simulink model "Task1"  (R2024a)
settings: Solver=VariableStepAuto  StartTime=0.0  StopTime=10.0  RelTol=1e-3
settings Model: Creator=artemzmailov  LastModifiedBy=artemzmailov

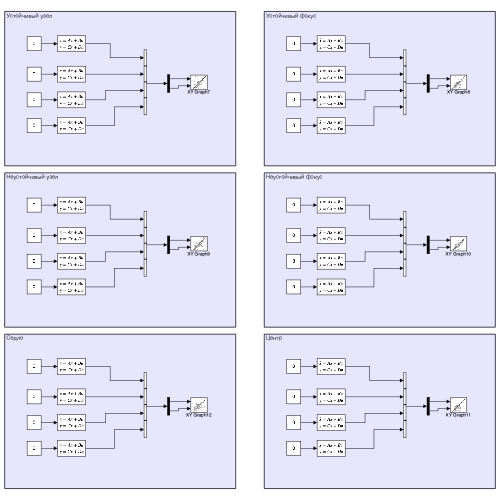
[thumbnail: Simulink's stored preview of the top-level diagram]
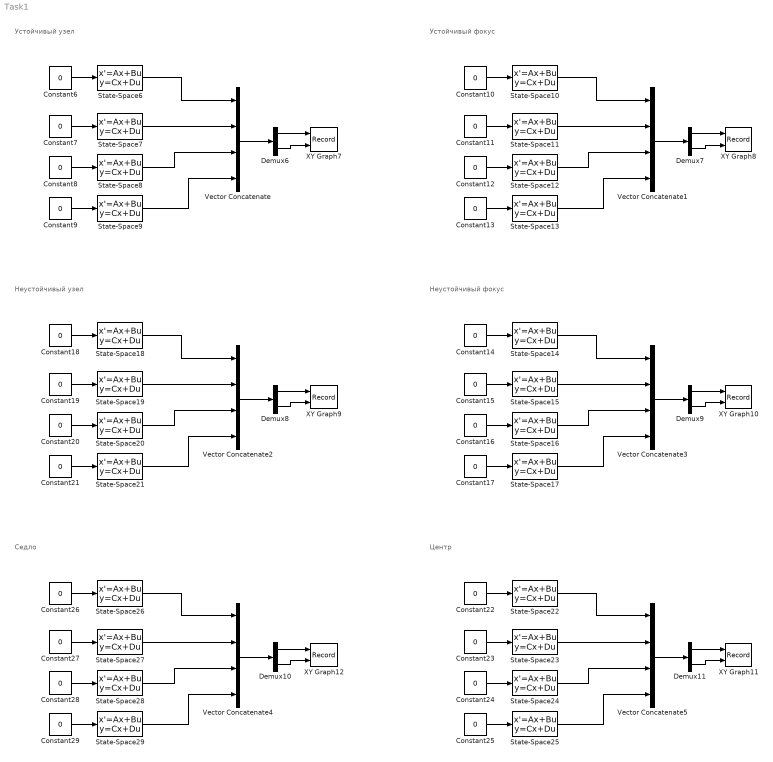
== system Task1 ==
  note: Устойчивый узел
  note: Устойчивый фокус
  note: Неустойчивый узел
  note: Неустойчивый фокус
  note: Седло
  note: Центр
  Constant{6..29} (24 alike) : Constant  Value=0
  Demux{6..11} (6 alike) : Demux  Outputs=2
  State-Space10 : StateSpace  A=[-1 -1; 2 -2]  B=[0;0]  C=[1 0; 0 1]  D=[0;0]  InitialCondition=[1;1]
  State-Space11 : StateSpace  A=[-1 0; 0 -2]  B=[0;0]  C=[1 0; 0 1]  D=[0;0]  InitialCondition=[-1;1]
  State-Space12 : StateSpace  A=[-1 0; 0 -2]  B=[0;0]  C=[1 0; 0 1]  D=[0;0]  InitialCondition=[3;-3]
  State-Space13 : StateSpace  A=[-1 0; 0 -2]  B=[0;0]  C=[1 0; 0 1]  D=[0;0]  InitialCondition=[-1;-1]
  State-Space14 : StateSpace  A=[1 -1; 2 2]  B=[0;0]  C=[1 0; 0 1]  D=[0;0]  InitialCondition=[1;1]
  State-Space15 : StateSpace  A=[1 -1; 2 2]  B=[0;0]  C=[1 0; 0 1]  D=[0;0]  InitialCondition=[-1;1]
  State-Space16 : StateSpace  A=[1 -1; 2 2]  B=[0;0]  C=[1 0; 0 1]  D=[0;0]  InitialCondition=[3;-3]
  State-Space17 : StateSpace  A=[1 -1; 2 2]  B=[0;0]  C=[1 0; 0 1]  D=[0;0]  InitialCondition=[-1;-1]
  State-Space18 : StateSpace  A=[1 0; 0 2]  B=[0;0]  C=[1 0; 0 1]  D=[0;0]  InitialCondition=[1;1]
  State-Space19 : StateSpace  A=[1 0; 0 2]  B=[0;0]  C=[1 0; 0 1]  D=[0;0]  InitialCondition=[-1;1]
  State-Space20 : StateSpace  A=[1 0; 0 2]  B=[0;0]  C=[1 0; 0 1]  D=[0;0]  InitialCondition=[0.5;-0.5]
  State-Space21 : StateSpace  A=[1 0; 0 2]  B=[0;0]  C=[1 0; 0 1]  D=[0;0]  InitialCondition=[-1;-1]
  State-Space22 : StateSpace  A=[0 -1; 1 0]  B=[0;0]  C=[1 0; 0 1]  D=[0;0]  InitialCondition=[1;1]
  State-Space23 : StateSpace  A=[0 -1; 1 0]  B=[0;0]  C=[1 0; 0 1]  D=[0;0]  InitialCondition=[-1;1]
  State-Space24 : StateSpace  A=[0 -1; 1 0]  B=[0;0]  C=[1 0; 0 1]  D=[0;0]  InitialCondition=[3;-3]
  State-Space25 : StateSpace  A=[0 -1; 1 0]  B=[0;0]  C=[1 0; 0 1]  D=[0;0]  InitialCondition=[-1;-1]
  State-Space26 : StateSpace  A=[1 0; 0 -2]  B=[0;0]  C=[1 0; 0 1]  D=[0;0]  InitialCondition=[1;1]
  State-Space27 : StateSpace  A=[1 0; 0 -2]  B=[0;0]  C=[1 0; 0 1]  D=[0;0]  InitialCondition=[-1;1]
  State-Space28 : StateSpace  A=[1 0; 0 -2]  B=[0;0]  C=[1 0; 0 1]  D=[0;0]  InitialCondition=[3;-3]
  State-Space29 : StateSpace  A=[1 0; 0 -2]  B=[0;0]  C=[1 0; 0 1]  D=[0;0]  InitialCondition=[-1;-1]
  State-Space6 : StateSpace  A=[-1 0; 0 -2]  B=[0;0]  C=[1 0; 0 1]  D=[0;0]  InitialCondition=[1;1]
  State-Space7 : StateSpace  A=[-1 0; 0 -2]  B=[0;0]  C=[1 0; 0 1]  D=[0;0]  InitialCondition=[-1;1]
  State-Space8 : StateSpace  A=[-1 0; 0 -2]  B=[0;0]  C=[1 0; 0 1]  D=[0;0]  InitialCondition=[3;-3]
  State-Space9 : StateSpace  A=[-1 0; 0 -2]  B=[0;0]  C=[1 0; 0 1]  D=[0;0]  InitialCondition=[-1;-1]
  Vector Concatenate{,1..5} (6 alike) : Concatenate  NumInputs=4
  XY Graph10 : Record  FileSettingsInternal="{\"entries\":[{\"content\":{\"excelSettings\":{\"content\":{},\"type\":\"Streamout.ExcelSettings\"}},\"type\":\"Streamout.FileSettingStorage\",\"uuid\":\"\"}],\"packageUris\":[\"http:\\/\\/schema.mathworks.com\\/mf0\\/streamout_blocks\\/R2020a\"],\"version\":\"1.0\"}"  Layout=[1 1]  SignalsInternal="{\"entries\":[{\"content\":{},\"type\":\"RecordBlkView.InputSignals\",\"uuid\":\"\"}],\"packageUris\":[\"http:\\/\\/schema.mathworks.com\\/mf0\\/streamout_blocks\\/R2020a\"],\"version\":\"1.0\"}"  VisualizationBindings="{\"xyplotplugin\":{\"info\":[{\"series\":[{\"bindingParametersList\":[{\"parameter\":\"X-Axis\",\"signalID\":2387,\"signalName\":\"Demux9:1(1)\"},{\"parameter\":\"Y-Axis\",\"signalID\":2392,\"signalName\":\"Demux9:2(1)\"}],\"seriesID\":0},{\"bindingParametersList\":[{\"parameter\":\"X-Axis\",\"signalID\":2442,\"signalName\":\"Demux9:1(2)\"},{\"parameter\":\"Y-Axis\",\"signalID\":2445,\"signalName\":\"Demux9:2(2)\"}],\"seriesID\":1},{\"bindingParametersList\":[{\"parameter\":\"X-Axis\",\"signalID\":2443,\"signalName\":\"Demux9:1(3)\"},{\"parameter\":\"Y-Axis\",\"signalID\":2446,\"signalName\":\"Demux9:2(3)\"}],\"seriesID\":2},{\"bindingParametersList\":[{\"parameter\":\"X-Axis\",\"signalID\":2444,\"signalName\":\"Demux9:1(4)\"},{\"parameter\":\"Y-Axis\",\"signalID\":2447,\"signalName\":\"Demux9:2(4)\"}],\"seriesID\":3}],\"subplotID\":1}]}}"  CompatibilityTag=XY
  XY Graph11 : Record  FileSettingsInternal="{\"entries\":[{\"content\":{\"excelSettings\":{\"content\":{},\"type\":\"Streamout.ExcelSettings\"}},\"type\":\"Streamout.FileSettingStorage\",\"uuid\":\"\"}],\"packageUris\":[\"http:\\/\\/schema.mathworks.com\\/mf0\\/streamout_blocks\\/R2020a\"],\"version\":\"1.0\"}"  Layout=[1 1]  SignalsInternal="{\"entries\":[{\"content\":{},\"type\":\"RecordBlkView.InputSignals\",\"uuid\":\"\"}],\"packageUris\":[\"http:\\/\\/schema.mathworks.com\\/mf0\\/streamout_blocks\\/R2020a\"],\"version\":\"1.0\"}"  VisualizationBindings="{\"xyplotplugin\":{\"info\":[{\"series\":[{\"bindingParametersList\":[{\"parameter\":\"X-Axis\",\"signalID\":2407,\"signalName\":\"Demux11:1(1)\"},{\"parameter\":\"Y-Axis\",\"signalID\":2412,\"signalName\":\"Demux11:2(1)\"}],\"seriesID\":0},{\"bindingParametersList\":[{\"parameter\":\"X-Axis\",\"signalID\":2454,\"signalName\":\"Demux11:1(2)\"},{\"parameter\":\"Y-Axis\",\"signalID\":2457,\"signalName\":\"Demux11:2(2)\"}],\"seriesID\":1},{\"bindingParametersList\":[{\"parameter\":\"X-Axis\",\"signalID\":2455,\"signalName\":\"Demux11:1(3)\"},{\"parameter\":\"Y-Axis\",\"signalID\":2458,\"signalName\":\"Demux11:2(3)\"}],\"seriesID\":2},{\"bindingParametersList\":[{\"parameter\":\"X-Axis\",\"signalID\":2456,\"signalName\":\"Demux11:1(4)\"},{\"parameter\":\"Y-Axis\",\"signalID\":2459,\"signalName\":\"Demux11:2(4)\"}],\"seriesID\":3}],\"subplotID\":1}]}}"  CompatibilityTag=XY
  XY Graph12 : Record  FileSettingsInternal="{\"entries\":[{\"content\":{\"excelSettings\":{\"content\":{},\"type\":\"Streamout.ExcelSettings\"}},\"type\":\"Streamout.FileSettingStorage\",\"uuid\":\"\"}],\"packageUris\":[\"http:\\/\\/schema.mathworks.com\\/mf0\\/streamout_blocks\\/R2020a\"],\"version\":\"1.0\"}"  Layout=[1 1]  SignalsInternal="{\"entries\":[{\"content\":{},\"type\":\"RecordBlkView.InputSignals\",\"uuid\":\"\"}],\"packageUris\":[\"http:\\/\\/schema.mathworks.com\\/mf0\\/streamout_blocks\\/R2020a\"],\"version\":\"1.0\"}"  VisualizationBindings="{\"xyplotplugin\":{\"info\":[{\"series\":[{\"bindingParametersList\":[{\"parameter\":\"X-Axis\",\"signalID\":2417,\"signalName\":\"Demux10:1(1)\"},{\"parameter\":\"Y-Axis\",\"signalID\":2422,\"signalName\":\"Demux10:2(1)\"}],\"seriesID\":0},{\"bindingParametersList\":[{\"parameter\":\"X-Axis\",\"signalID\":2460,\"signalName\":\"Demux10:1(2)\"},{\"parameter\":\"Y-Axis\",\"signalID\":2463,\"signalName\":\"Demux10:2(2)\"}],\"seriesID\":1},{\"bindingParametersList\":[{\"parameter\":\"X-Axis\",\"signalID\":2461,\"signalName\":\"Demux10:1(3)\"},{\"parameter\":\"Y-Axis\",\"signalID\":2464,\"signalName\":\"Demux10:2(3)\"}],\"seriesID\":2},{\"bindingParametersList\":[{\"parameter\":\"X-Axis\",\"signalID\":2462,\"signalName\":\"Demux10:1(4)\"},{\"parameter\":\"Y-Axis\",\"signalID\":2465,\"signalName\":\"Demux10:2(4)\"}],\"seriesID\":3}],\"subplotID\":1}]}}"  CompatibilityTag=XY
  XY Graph7 : Record  FileSettingsInternal="{\"entries\":[{\"content\":{\"excelSettings\":{\"content\":{},\"type\":\"Streamout.ExcelSettings\"}},\"type\":\"Streamout.FileSettingStorage\",\"uuid\":\"\"}],\"packageUris\":[\"http:\\/\\/schema.mathworks.com\\/mf0\\/streamout_blocks\\/R2020a\"],\"version\":\"1.0\"}"  Layout=[1 1]  SignalsInternal="{\"entries\":[{\"content\":{},\"type\":\"RecordBlkView.InputSignals\",\"uuid\":\"\"}],\"packageUris\":[\"http:\\/\\/schema.mathworks.com\\/mf0\\/streamout_blocks\\/R2020a\"],\"version\":\"1.0\"}"  VisualizationBindings="{\"xyplotplugin\":{\"info\":[{\"series\":[{\"bindingParametersList\":[{\"parameter\":\"X-Axis\",\"signalID\":2427,\"signalName\":\"Demux6:1(1)\"},{\"parameter\":\"Y-Axis\",\"signalID\":2432,\"signalName\":\"Demux6:2(1)\"},{\"parameter\":\"X-Axis\",\"signalID\":2427,\"signalName\":\"Demux6:1(1)\"},{\"parameter\":\"Y-Axis\",\"signalID\":2432,\"signalName\":\"Demux6:2(1)\"},{\"parameter\":\"X-Axis\",\"signalID\":2427,\"signalName\":\"Demux6:1(1)\"},{\"parameter\":\"Y-Axis\",\"signalID\":2432,\"signalName\":\"Demux6:2(1)\"},{\"parameter\":\"X-Axis\",\"signalID\":2427,\"signalName\":\"Demux6:1(1)\"},{\"parameter\":\"Y-Axis\",\"signalID\":2432,\"signalName\":\"Demux6:2(1)\"},{\"parameter\":\"X-Axis\",\"signalID\":2427,\"signalName\":\"Demux6:1(1)\"},{\"parameter\":\"Y-Axis\",\"signalID\":2432,\"signalName\":\"Demux6:2(1)\"},{\"parameter\":\"X-Axis\",\"signalID\":2427,\"signalName\":\"Demux6:1(1)\"},{\"parameter\":\"Y-Axis\",\"signalID\":2432,\"signalName\":\"Demux6:2(1)\"},{\"parameter\":\"X-Axis\",\"signalID\":2427,\"signalName\":\"Demux6:1(1)\"},{\"parameter\":\"Y-Axis\",\"signalID\":2432,\"signalName\":\"Demux6:2(1)\"},{\"parameter\":\"X-Axis\",\"signalID\":2427,\"signalName\":\"Demux6:1(1)\"},{\"parameter\":\"Y-Axis\",\"signalID\":2432,\"signalName\":\"Demux6:2(1)\"},{\"parameter\":\"X-Axis\",\"signalID\":2427,\"signalName\":\"Demux6:1(1)\"},{\"parameter\":\"Y-Axis\",\"signalID\":2432,\"signalName\":\"Demux6:2(1)\"},{\"parameter\":\"X-Axis\",\"signalID\":2427,\"signalName\":\"Demux6:1(1)\"},{\"parameter\":\"Y-Axis\",\"signalID\":2432,\"signalName\":\"Demux6:2(1)\"},{\"parameter\":\"X-Axis\",\"signalID\":2427,\"signalName\":\"Demux6:1(1)\"},{\"parameter\":\"Y-Axis\",\"signalID\":2432,\"signalName\":\"Demux6:2(1)\"},{\"parameter\":\"X-Axis\",\"signalID\":2427,\"signalName\":\"Demux6:1(1)\"},{\"parameter\":\"Y-Axis\",\"signalID\":2432,\"signalName\":\"Demux6:2(1)\"},{\"parameter\":\"X-Axis\",\"signalID\":2427,\"signalName\":\"Demux6:1(1)\"},{\"parameter\":\"Y-Axis\",\"signalID\":2432,\"signalName\":\"Demux6:2(1)\"},{\"parameter\":\"X-Axis\",\"signalID\":2427,\"signalName\":\"Demux6:1(1)\"},{\"parameter\":\"Y-Axis\",\"signalID\":2432,\"signalName\":\"Demux6:2(1)\"},{\"parameter\":\"X-Axis\",\"signalID\":2427,\"signalName\":\"Demux6:1(1)\"},{\"parameter\":\"Y-Axis\",\"signalID\":2432,\"signalName\":\"Demux6:2(1)\"},{\"parameter\":\"X-Axis\",\"signalID\":2427,\"signalName\":\"Demux6:1(1)\"},{\"parameter\":\"Y-Axis\",\"signalID\":2432,\"signalName\":\"Demux6:2(1)\"}],\"seriesID\":0},{\"bindingParametersList\":[{\"parameter\":\"X-Axis\",\"signalID\":2466,\"signalName\":\"Demux6:1(2)\"},{\"parameter\":\"Y-Axis\",\"signalID\":2469,\"signalName\":\"Demux6:2(2)\"},{\"parameter\":\"X-Axis\",\"signalID\":2466,\"signalName\":\"Demux6:1(2)\"},{\"parameter\":\"Y-Axis\",\"signalID\":2469,\"signalName\":\"Demux6:2(2)\"},{\"parameter\":\"X-Axis\",\"signalID\":2466,\"signalName\":\"Demux6:1(2)\"},{\"parameter\":\"Y-Axis\",\"signalID\":2469,\"signalName\":\"Demux6:2(2)\"},{\"parameter\":\"X-Axis\",\"signalID\":2466,\"signalName\":\"Demux6:1(2)\"},{\"parameter\":\"Y-Axis\",\"signalID\":2469,\"signalName\":\"Demux6:2(2)\"},{\"parameter\":\"X-Axis\",\"signalID\":2466,\"signalName\":\"Demux6:1(2)\"},{\"parameter\":\"Y-Axis\",\"signalID\":2469,\"signalName\":\"Demux6:2(2)\"},{\"parameter\":\"X-Axis\",\"signalID\":2466,\"signalName\":\"Demux6:1(2)\"},{\"parameter\":\"Y-Axis\",\"signalID\":2469,\"signalName\":\"Demux6:2(2)\"},{\"parameter\":\"X-Axis\",\"signalID\":2466,\"signalName\":\"Demux6:1(2)\"},{\"parameter\":\"Y-Axis\",\"signalID\":2469,\"signalName\":\"Demux6:2(2)\"},{\"parameter\":\"X-Axis\",\"signalID\":2466,\"signalName\":\"Demux6:1(2)\"},{\"parameter\":\"Y-Axis\",\"signalID\":2469,\"signalName\":\"Demux6:2(2)\"},{\"parameter\":\"X-Axis\",\"signalID\":2466,\"signalName\":\"Demux6:1(2)\"},{\"parameter\":\"Y-Axis\",\"signalID\":2469,\"signalName\":\"Demux6:2(2)\"},{\"parameter\":\"X-Axis\",\"signalID\":2466,\"signalName\":\"Demux6:1(2)\"},{\"parameter\":\"Y-Axis\",\"signalID\":2469,\"signalName\":\"Demux6:2(2)\"},{\"parameter\":\"X-Axis\",\"signalID\":2466,\"signalName\":\"Demux6:1(2)\"},{\"parameter\":\"Y-Axis\",\"signalID\":2469,\"signalName\":\"Demux6:2(2)\"},{\"parameter\":\"X-Axis\",\"signalID\":2466,\"signalName\":\"Demux6:1(2)\"},{\"parameter\":\"Y-Axis\",\"signalID\":2469,\"signalName\":\"Demux6:2(2)\"},{\"parameter\":\"X-Axis\",\"signalID\":2466,\"signalName\":\"Demux6:1(2)\"},{\"parameter\":\"Y-Axis\",\"signalID\":2469,\"signalName\":\"Demux6:2(2)\"},{\"parameter\":\"X-Axis\",\"signalID\":2466,\"signalName\":\"Demux6:1(2)\"},{\"parameter\":\"Y-Axis\",\"signalID\":2469,\"signalName\":\"Demux6:2(2)\"},{\"parameter\":\"X-Axis\",\"signalID\":2466,\"signalName\":\"Demux6:1(2)\"},{\"parameter\":\"Y-Axis\",\"signalID\":2469,\"signalName\":\"Demux6:2(2)\"}],\"seriesID\":1},{\"bindingParametersList\":[{\"parameter\":\"X-Axis\",\"signalID\":2467,\"signalName\":\"Demux6:1(3)\"},{\"parameter\":\"Y-Axis\",\"signalID\":2470,\"signalName\":\"Demux6:2(3)\"},{\"parameter\":\"X-Axis\",\"signalID\":2467,\"signalName\":\"Demux6:1(3)\"},{\"parameter\":\"Y-Axis\",\"signalID\":2470,\"signalName\":\"Demux6:2(3)\"},{\"parameter\":\"X-Axis\",\"signalID\":2467,\"signalName\":\"Demux6:1(3)\"},{\"parameter\":\"Y-Axis\",\"signalID\":2470,\"signalName\":\"Demux6:2(3)\"},{\"parameter\":\"X-Axis\",\"signalID\":2467,\"signalName\":\"Demux6:1(3)\"},{\"parameter\":\"Y-Axis\",\"signalID\":2470,\"signalName\":\"Demux6:2(3)\"},{\"parameter\":\"X-Axis\",\"signalID\":2467,\"signalName\":\"Demux6:1(3)\"},{\"parameter\":\"Y-Axis\",\"signalID\":2470,\"signalName\":\"Demux6:2(3)\"},{\"parameter\":\"X-Axis\",\"signalID\":2467,\"signalName\":\"Demux6:1(3)\"},{\"parameter\":\"Y-Axis\",\"signalID\":2470,\"signalName\":\"Demux6:2(3)\"},{\"parameter\":\"X-Axis\",\"signalID\":2467,\"signalName\":\"Demux6:1(3)\"},{\"parameter\":\"Y-Axis\",\"signalID\":2470,\"signalName\":\"Demux6:2(3)\"},{\"parameter\":\"X-Axis\",\"signalID\":2467,\"signalName\":\"Demux6:1(3)\"},{\"parameter\":\"Y-Axis\",\"signalID\":2470,\"signalName\":\"Demux6:2(3)\"},{\"parameter\":\"X-Axis\",\"signalID\":2467,\"signalName\":\"Demux6:1(3)\"},{\"parameter\":\"Y-Axis\",\"signalID\":2470,\"signalName\":\"Demux6:2(3)\"},{\"parameter\":\"X-Axis\",\"signalID\":2467,\"signalName\":\"Demux6:1(3)\"},{\"parameter\":\"Y-Axis\",\"signalID\":2470,\"signalName\":\"Demux6:2(3)\"},{\"parameter\":\"X-Axis\",\"signalID\":2467,\"signalName\":\"Demux6:1(3)\"},{\"parameter\":\"Y-Axis\",\"signalID\":2470,\"signalName\":\"Demux6:2(3)\"},{\"parameter\":\"X-Axis\",\"signalID\":2467,\"signalName\":\"Demux6:1(3)\"},{\"parameter\":\"Y-Axis\",\"signalID\":2470,\"signalName\":\"Demux6:2(3)\"},{\"parameter\":\"X-Axis\",\"signalID\":2467,\"signalName\":\"Demux6:1(3)\"},{\"parameter\":\"Y-Axis\",\"signalID\":2470,\"signalName\":\"Demux6:2(3)\"},{\"parameter\":\"X-Axis\",\"signalID\":2467,\"signalName\":\"Demux6:1(3)\"},{\"parameter\":\"Y-Axis\",\"signalID\":2470,\"signalName\":\"Demux6:2(3)\"}],\"seriesID\":2},{\"bindingParametersList\":[{\"parameter\":\"X-Axis\",\"signalID\":2468,\"signalName\":\"Demux6:1(4)\"},{\"parameter\":\"Y-Axis\",\"signalID\":2471,\"signalName\":\"Demux6:2(4)\"},{\"parameter\":\"X-Axis\",\"signalID\":2468,\"signalName\":\"Demux6:1(4)\"},{\"parameter\":\"Y-Axis\",\"signalID\":2471,\"signalName\":\"Demux6:2(4)\"},{\"parameter\":\"X-Axis\",\"signalID\":2468,\"signalName\":\"Demux6:1(4)\"},{\"parameter\":\"Y-Axis\",\"signalID\":2471,\"signalName\":\"Demux6:2(4)\"},{\"parameter\":\"X-Axis\",\"signalID\":2468,\"signalName\":\"Demux6:1(4)\"},{\"parameter\":\"Y-Axis\",\"signalID\":2471,\"signalName\":\"Demux6:2(4)\"},{\"parameter\":\"X-Axis\",\"signalID\":2468,\"signalName\":\"Demux6:1(4)\"},{\"parameter\":\"Y-Axis\",\"signalID\":2471,\"signalName\":\"Demux6:2(4)\"},{\"parameter\":\"X-Axis\",\"signalID\":2468,\"signalName\":\"Demux6:1(4)\"},{\"parameter\":\"Y-Axis\",\"signalID\":2471,\"signalName\":\"Demux6:2(4)\"},{\"parameter\":\"X-Axis\",\"signalID\":2468,\"signalName\":\"Demux6:1(4)\"},{\"parameter\":\"Y-Axis\",\"signalID\":2471,\"signalName\":\"Demux6:2(4)\"},{\"parameter\":\"X-Axis\",\"signalID\":2468,\"signalName\":\"Demux6:1(4)\"},{\"parameter\":\"Y-Axis\",\"signalID\":2471,\"signalName\":\"Demux6:2(4)\"}],\"seriesID\":3}],\"subplotID\":1}]}}"  CompatibilityTag=XY
  XY Graph8 : Record  FileSettingsInternal="{\"entries\":[{\"content\":{\"excelSettings\":{\"content\":{},\"type\":\"Streamout.ExcelSettings\"}},\"type\":\"Streamout.FileSettingStorage\",\"uuid\":\"\"}],\"packageUris\":[\"http:\\/\\/schema.mathworks.com\\/mf0\\/streamout_blocks\\/R2020a\"],\"version\":\"1.0\"}"  Layout=[1 1]  SignalsInternal="{\"entries\":[{\"content\":{},\"type\":\"RecordBlkView.InputSignals\",\"uuid\":\"\"}],\"packageUris\":[\"http:\\/\\/schema.mathworks.com\\/mf0\\/streamout_blocks\\/R2020a\"],\"version\":\"1.0\"}"  VisualizationBindings="{\"xyplotplugin\":{\"info\":[{\"series\":[{\"bindingParametersList\":[{\"parameter\":\"X-Axis\",\"signalID\":2377,\"signalName\":\"Demux7:1(1)\"},{\"parameter\":\"Y-Axis\",\"signalID\":2382,\"signalName\":\"Demux7:2(1)\"}],\"seriesID\":0},{\"bindingParametersList\":[{\"parameter\":\"X-Axis\",\"signalID\":2436,\"signalName\":\"Demux7:1(2)\"},{\"parameter\":\"Y-Axis\",\"signalID\":2439,\"signalName\":\"Demux7:2(2)\"}],\"seriesID\":1},{\"bindingParametersList\":[{\"parameter\":\"X-Axis\",\"signalID\":2437,\"signalName\":\"Demux7:1(3)\"},{\"parameter\":\"Y-Axis\",\"signalID\":2440,\"signalName\":\"Demux7:2(3)\"}],\"seriesID\":2},{\"bindingParametersList\":[{\"parameter\":\"X-Axis\",\"signalID\":2438,\"signalName\":\"Demux7:1(4)\"},{\"parameter\":\"Y-Axis\",\"signalID\":2441,\"signalName\":\"Demux7:2(4)\"}],\"seriesID\":3}],\"subplotID\":1}]}}"  CompatibilityTag=XY
  XY Graph9 : Record  FileSettingsInternal="{\"entries\":[{\"content\":{\"excelSettings\":{\"content\":{},\"type\":\"Streamout.ExcelSettings\"}},\"type\":\"Streamout.FileSettingStorage\",\"uuid\":\"\"}],\"packageUris\":[\"http:\\/\\/schema.mathworks.com\\/mf0\\/streamout_blocks\\/R2020a\"],\"version\":\"1.0\"}"  Layout=[1 1]  SignalsInternal="{\"entries\":[{\"content\":{\"signals\":[{\"content\":{\"blockPath\":[],\"dimensions\":[4],\"domain\":\"\",\"hasChildren\":true,\"lineColor\":\"#a2142f\",\"lineWidth\":2,\"port\":1,\"sid\":[\"\"],\"signalID\":1,\"signalName\":\"Demux7:1\"},\"type\":\"RecordBlkView.Signal\",\"uuid\":\"\"},{\"content\":{\"blockPath\":[],\"channel\":[1],\"dimensions\":[4],\"domain\":\"\",\"lineColor\":\"#7e2f8e\",\"lineWidth\":2,\"parentID\":1,\"port\":1,\"sid\":[\"\"],\"signalID\":2,\"signalName\":\"Demux7:1\"},\"type\":\"RecordBlkView.Signal\",\"uuid\":\"\"},{\"content\":{\"blockPath\":[],\"dimensions\":[4],\"domain\":\"\",\"hasChildren\":true,\"lineColor\":\"#ff6929\",\"lineWidth\":2,\"port\":2,\"sid\":[\"\"],\"signalID\":3,\"signalName\":\"Demux7:2\"},\"type\":\"RecordBlkView.Signal\",\"uuid\":\"\"},{\"content\":{\"blockPath\":[],\"channel\":[1],\"dimensions\":[4],\"domain\":\"\",\"lineColor\":\"#4dbeee\",\"lineWidth\":2,\"parentID\":3,\"port\":2,\"sid\":[\"\"],\"signalID\":4,\"signalName\":\"Demux7:2\"},\"type\":\"RecordBlkView.Signal\",\"uuid\":\"\"},{\"content\":{\"blockPath\":[],\"dimensions\":[4],\"domain\":\"\",\"hasChildren\":true,\"lineColor\":\"#64d413\",\"lineWidth\":2,\"port\":1,\"sid\":[\"\"],\"signalID\":5,\"signalName\":\"Demux9:1\"},\"type\":\"RecordBlkView.Signal\",\"uuid\":\"\"},{\"content\":{\"blockPath\":[],\"channel\":[1],\"dimensions\":[4],\"domain\":\"\",\"lineColor\":\"#7e2f8e\",\"lineWidth\":2,\"parentID\":5,\"port\":1,\"sid\":[\"\"],\"signalID\":6,\"signalName\":\"Demux9:1\"},\"type\":\"RecordBlkView.Signal\",\"uuid\":\"\"},{\"content\":{\"blockPath\":[],\"dimensions\":[4],\"domain\":\"\",\"hasChildren\":true,\"lineColor\":\"#fe330a\",\"lineWidth\":2,\"port\":2,\"sid\":[\"\"],\"signalID\":7,\"signalName\":\"Demux9:2\"},\"type\":\"RecordBlkView.Signal\",\"uuid\":\"\"},{\"content\":{\"blockPath\":[],\"channel\":[1],\"dimensions\":[4],\"domain\":\"\",\"lineColor\":\"#4dbeee\",\"lineWidth\":2,\"parentID\":7,\"port\":2,\"sid\":[\"\"],\"signalID\":8,\"signalName\":\"Demux9:2\"},\"type\":\"RecordBlkView.Signal\",\"uuid\":\"\"},{\"content\":{\"blockPath\":[],\"dimensions\":[4],\"domain\":\"\",\"hasChildren\":true,\"lineColor\":\"#0072bd\",\"lineWidth\":2,\"port\":1,\"sid\":[\"\"],\"signalID\":9,\"signalName\":\"Demux8:1\"},\"type\":\"RecordBlkView.Signal\",\"uuid\":\"\"},{\"content\":{\"blockPath\":[],\"channel\":[1],\"dimensions\":[4],\"domain\":\"\",\"lineColor\":\"#7e2f8e\",\"lineWidth\":2,\"parentID\":9,\"plots\":[ 1 ],\"port\":1,\"sid\":[\"\"],\"signalID\":10,\"signalName\":\"Demux8:1\"},\"type\":\"RecordBlkView.Signal\",\"uuid\":\"\"},{\"content\":{\"blockPath\":[],\"dimensions\":[4],\"domain\":\"\",\"hasChildren\":true,\"lineColor\":\"#edb120\",\"lineWidth\":2,\"port\":2,\"sid\":[\"\"],\"signalID\":11,\"signalName\":\"Demux8:2\"},\"type\":\"RecordBlkView.Signal\",\"uuid\":\"\"},{\"content\":{\"blockPath\":[],\"channel\":[1],\"dimensions\":[4],\"domain\":\"\",\"lineColor\":\"#4dbeee\",\"lineWidth\":2,\"parentID\":11,\"plots\":[ 1 ],\"port\":2,\"sid\":[\"\"],\"signalID\":12,\"signalName\":\"Demux8:2\"},\"type\":\"RecordBlkView.Signal\",\"uuid\":\"\"},{\"content\":{\"blockPath\":[],\"dimensions\":[4],\"domain\":\"\",\"hasChildren\":true,\"lineColor\":\"#77ac30\",\"lineWidth\":2,\"port\":1,\"sid\":[\"\"],\"signalID\":13,\"signalName\":\"Demux11:1\"},\"type\":\"RecordBlkView.Signal\",\"uuid\":\"\"},{\"content\":{\"blockPath\":[],\"channel\":[1],\"dimensions\":[4],\"domain\":\"\",\"lineColor\":\"#7e2f8e\",\"lineWidth\":2,\"parentID\":13,\"port\":1,\"sid\":[\"\"],\"signalID\":14,\"signalName\":\"Demux11:1\"},\"type\":\"RecordBlkView.Signal\",\"uuid\":\"\"},{\"content\":{\"blockPath\":[],\"dimensions\":[4],\"domain\":\"\",\"hasChildren\":true,\"lineColor\":\"#a2142f\",\"lineWidth\":2,\"port\":2,\"sid\":[\"\"],\"signalID\":15,\"signalName\":\"Demux11:2\"},\"type\":\"RecordBlkView.Signal\",\"uuid\":\"\"},{\"content\":{\"blockPath\":[],\"channel\":[1],\"dimensions\":[4],\"domain\":\"\",\"lineColor\":\"#4dbeee\",\"lineWidth\":2,\"parentID\":15,\"port\":2,\"sid\":[\"\"],\"signalID\":16,\"signalName\":\"Demux11:2\"},\"type\":\"RecordBlkView.Signal\",\"uuid\":\"\"},{\"content\":{\"blockPath\":[],\"dimensions\":[4],\"domain\":\"\",\"hasChildren\":true,\"lineColor\":\"#ff6929\",\"lineWidth\":2,\"port\":1,\"sid\":[\"\"],\"signalID\":17,\"signalName\":\"Demux10:1\"},\"type\":\"RecordBlkView.Signal\",\"uuid\":\"\"},{\"content\":{\"blockPath\":[],\"channel\":[1],\"dimensions\":[4],\"domain\":\"\",\"lineColor\":\"#7e2f8e\",\"lineWidth\":2,\"parentID\":17,\"port\":1,\"sid\":[\"\"],\"signalID\":18,\"signalName\":\"Demux10:1\"},\"type\":\"RecordBlkView.Signal\",\"uuid\":\"\"},{\"content\":{\"blockPath\":[],\"dimensions\":[4],\"domain\":\"\",\"hasChildren\":true,\"lineColor\":\"#64d413\",\"lineWidth\":2,\"port\":2,\"sid\":[\"\"],\"signalID\":19,\"signalName\":\"Demux10:2\"},\"type\":\"RecordBlkView.Signal\",\"uuid\":\"\"},{\"content\":{\"blockPath\":[],\"channel\":[1],\"dimensions\":[4],\"domain\":\"\",\"lineColor\":\"#4dbeee\",\"lineWidth\":2,\"parentID\":19,\"port\":2,\"sid\":[\"\"],\"signalID\":20,\"signalName\":\"Demux10:2\"},\"type\":\"RecordBlkView.Signal\",\"uuid\":\"\"},{\"content\":{\"blockPath\":[],\"dimensions\":[4],\"domain\":\"\",\"hasChildren\":true,\"lineColor\":\"#fe330a\",\"lineWidth\":2,\"port\":1,\"sid\":[\"\"],\"signalID\":21,\"signalName\":\"Demux6:1\"},\"type\":\"RecordBlkView.Signal\",\"uuid\":\"\"},{\"content\":{\"blockPath\":[],\"channel\":[1],\"dimensions\":[4],\"domain\":\"\",\"lineColor\":\"#7e2f8e\",\"lineWidth\":2,\"parentID\":21,\"port\":1,\"sid\":[\"\"],\"signalID\":22,\"signalName\":\"Demux6:1\"},\"type\":\"RecordBlkView.Signal\",\"uuid\":\"\"},{\"content\":{\"blockPath\":[],\"dimensions\":[4],\"domain\":\"\",\"hasChildren\":true,\"lineColor\":\"#0072bd\",\"lineWidth\":2,\"port\":2,\"sid\":[\"\"],\"signalID\":23,\"signalName\":\"Demux6:2\"},\"type\":\"RecordBlkView.Signal\",\"uuid\":\"\"},{\"content\":{\"blockPath\":[],\"channel\":[1],\"dimensions\":[4],\"domain\":\"\",\"lineColor\":\"#4dbeee\",\"lineWidth\":2,\"parentID\":23,\"port\":2,\"sid\":[\"\"],\"signalID\":24,\"signalName\":\"Demux6:2\"},\"type\":\"RecordBlkView.Signal\",\"uuid\":\"\"},{\"content\":{\"blockPath\":[],\"channel\":[2],\"dimensions\":[4],\"domain\":\"\",\"lineColor\":\"#ff6929\",\"lineWidth\":2,\"parentID\":1,\"port\":1,\"sid\":[\"\"],\"signalID\":25,\"signalName\":\"Demux7:1\"},\"type\":\"RecordBlkView.Signal\",\"uuid\":\"\"},{\"content\":{\"blockPath\":[],\"channel\":[3],\"dimensions\":[4],\"domain\":\"\",\"lineColor\":\"#b746ff\",\"lineWidth\":2,\"parentID\":1,\"port\":1,\"sid\":[\"\"],\"signalID\":26,\"signalName\":\"Demux7:1\"},\"type\":\"RecordBlkView.Signal\",\"uuid\":\"\"},{\"content\":{\"blockPath\":[],\"channel\":[4],\"dimensions\":[4],\"domain\":\"\",\"lineColor\":\"#64d413\",\"lineWidth\":2,\"parentID\":1,\"port\":1,\"sid\":[\"\"],\"signalID\":27,\"signalName\":\"Demux7:1\"},\"type\":\"RecordBlkView.Signal\",\"uuid\":\"\"},{\"content\":{\"blockPath\":[],\"channel\":[2],\"dimensions\":[4],\"domain\":\"\",\"lineColor\":\"#ff13a6\",\"lineWidth\":2,\"parentID\":3,\"port\":2,\"sid\":[\"\"],\"signalID\":28,\"signalName\":\"Demux7:2\"},\"type\":\"RecordBlkView.Signal\",\"uuid\":\"\"},{\"content\":{\"blockPath\":[],\"channel\":[3],\"dimensions\":[4],\"domain\":\"\",\"lineColor\":\"#fe330a\",\"lineWidth\":2,\"parentID\":3,\"port\":2,\"sid\":[\"\"],\"signalID\":29,\"signalName\":\"Demux7:2\"},\"type\":\"RecordBlkView.Signal\",\"uuid\":\"\"},{\"content\":{\"blockPath\":[],\"channel\":[4],\"dimensions\":[4],\"domain\":\"\",\"lineColor\":\"#22b573\",\"lineWidth\":2,\"parentID\":3,\"port\":2,\"sid\":[\"\"],\"signalID\":30,\"signalName\":\"Demux7:2\"},\"type\":\"RecordBlkView.Signal\",\"uuid\":\"\"},{\"content\":{\"blockPath\":[],\"channel\":[2],\"dimensions\":[4],\"domain\":\"\",\"lineColor\":\"#ff6929\",\"lineWidth\":2,\"parentID\":5,\"port\":1,\"sid\":[\"\"],\"signalID\":31,\"signalName\":\"Demux9:1\"},\"type\":\"RecordBlkView.Signal\",\"uuid\":\"\"},{\"content\":{\"blockPath\":[],\"channel\":[3],\"dimensions\":[4],\"domain\":\"\",\"lineColor\":\"#b746ff\",\"lineWidth\":2,\"parentID\":5,\"port\":1,\"sid\":[\"\"],\"signalID\":32,\"signalName\":\"Demux9:1\"},\"type\":\"RecordBlkView.Signal\",\"uuid\":\"\"},{\"content\":{\"blockPath\":[],\"channel\":[4],\"dimensions\":[4],\"domain\":\"\",\"lineColor\":\"#64d413\",\"lineWidth\":2,\"parentID\":5,\"port\":1,\"sid\":[\"\"],\"signalID\":33,\"signalName\":\"Demux9:1\"},\"type\":\"RecordBlkView.Signal\",\"uuid\":\"\"},{\"content\":{\"blockPath\":[],\"channel\":[2],\"dimensions\":[4],\"domain\":\"\",\"lineColor\":\"#ff13a6\",\"lineWidth\":2,\"parentID\":7,\"port\":2,\"sid\":[\"\"],\"signalID\":34,\"signalName\":\"Demux9:2\"},\"type\":\"RecordBlkView.Signal\",\"uuid\":\"\"},{\"content\":{\"blockPath\":[],\"channel\":[3],\"dimensions\":[4],\"domain\":\"\",\"lineColor\":\"#fe330a\",\"lineWidth\":2,\"parentID\":7,\"port\":2,\"sid\":[\"\"],\"signalID\":35,\"signalName\":\"Demux9:2\"},\"type\":\"RecordBlkView.Signal\",\"uuid\":\"\"},{\"content\":{\"blockPath\":[],\"channel\":[4],\"dimensions\":[4],\"domain\":\"\",\"lineColor\":\"#22b573\",\"lineWidth\":2,\"parentID\":7,\"port\":2,\"sid\":[\"\"],\"signalID\":36,\"signalName\":\"Demux9:2\"},\"type\":\"RecordBlkView.Signal\",\"uuid\":\"\"},{\"content\":{\"blockPath\":[],\"channel\":[2],\"dimensions\":[4],\"domain\":\"\",\"lineColor\":\"#ff6929\",\"lineWidth\":2,\"parentID\":9,\"plots\":[ 1 ],\"port\":1,\"sid\":[\"\"],\"signalID\":37,\"signalName\":\"Demux8:1\"},\"type\":\"RecordBlkView.Signal\",\"uuid\":\"\"},{\"content\":{\"blockPath\":[],\"channel\":[3],\"dimensions\":[4],\"domain\":\"\",\"lineColor\":\"#b746ff\",\"lineWidth\":2,\"parentID\":9,\"plots\":[ 1 ],\"port\":1,\"sid\":[\"\"],\"signalID\":38,\"signalName\":\"Demux8:1\"},\"type\":\"RecordBlkView.Signal\",\"uuid\":\"\"},{\"content\":{\"blockPath\":[],\"channel\":[4],\"dimensions\":[4],\"domain\":\"\",\"lineColor\":\"#64d413\",\"lineWidth\":2,\"parentID\":9,\"plots\":[ 1 ],\"port\":1,\"sid\":[\"\"],\"signalID\":39,\"signalName\":\"Demux8:1\"},\"type\":\"RecordBlkView.Signal\",\"uuid\":\"\"},{\"content\":{\"blockPath\":[],\"channel\":[2],\"dimensions\":[4],\"domain\":\"\",\"lineColor\":\"#ff13a6\",\"lineWidth\":2,\"parentID\":11,\"plots\":[ 1 ],\"port\":2,\"sid\":[\"\"],\"signalID\":40,\"signalName\":\"Demux8:2\"},\"type\":\"RecordBlkView.Signal\",\"uuid\":\"\"},{\"content\":{\"blockPath\":[],\"channel\":[3],\"dimensions\":[4],\"domain\":\"\",\"lineColor\":\"#fe330a\",\"lineWidth\":2,\"parentID\":11,\"plots\":[ 1 ],\"port\":2,\"sid\":[\"\"],\"signalID\":41,\"signalName\":\"Demux8:2\"},\"type\":\"RecordBlkView.Signal\",\"uuid\":\"\"},{\"content\":{\"blockPath\":[],\"channel\":[4],\"dimensions\":[4],\"domain\":\"\",\"lineColor\":\"#22b573\",\"lineWidth\":2,\"parentID\":11,\"plots\":[ 1 ],\"port\":2,\"sid\":[\"\"],\"signalID\":42,\"signalName\":\"Demux8:2\"},\"type\":\"RecordBlkView.Signal\",\"uuid\":\"\"},{\"content\":{\"blockPath\":[],\"channel\":[2],\"dimensions\":[4],\"domain\":\"\",\"lineColor\":\"#ff6929\",\"lineWidth\":2,\"parentID\":13,\"port\":1,\"sid\":[\"\"],\"signalID\":43,\"signalName\":\"Demux11:1\"},\"type\":\"RecordBlkView.Signal\",\"uuid\":\"\"},{\"content\":{\"blockPath\":[],\"channel\":[3],\"dimensions\":[4],\"domain\":\"\",\"lineColor\":\"#b746ff\",\"lineWidth\":2,\"parentID\":13,\"port\":1,\"sid\":[\"\"],\"signalID\":44,\"signalName\":\"Demux11:1\"},\"type\":\"RecordBlkView.Signal\",\"uuid\":\"\"},{\"content\":{\"blockPath\":[],\"channel\":[4],\"dimensions\":[4],\"domain\":\"\",\"lineColor\":\"#64d413\",\"lineWidth\":2,\"parentID\":13,\"port\":1,\"sid\":[\"\"],\"signalID\":45,\"signalName\":\"Demux11:1\"},\"type\":\"RecordBlkView.Signal\",\"uuid\":\"\"},{\"content\":{\"blockPath\":[],\"channel\":[2],\"dimensions\":[4],\"domain\":\"\",\"lineColor\":\"#ff13a6\",\"lineWidth\":2,\"parentID\":15,\"port\":2,\"sid\":[\"\"],\"signalID\":46,\"signalName\":\"Demux11:2\"},\"type\":\"RecordBlkView.Signal\",\"uuid\":\"\"},{\"content\":{\"blockPath\":[],\"channel\":[3],\"dimensions\":[4],\"domain\":\"\",\"lineColor\":\"#fe330a\",\"lineWidth\":2,\"parentID\":15,\"port\":2,\"sid\":[\"\"],\"signalID\":47,\"signalName\":\"Demux11:2\"},\"type\":\"RecordBlkView.Signal\",\"uuid\":\"\"},{\"content\":{\"blockPath\":[],\"channel\":[4],\"dimensions\":[4],\"domain\":\"\",\"lineColor\":\"#22b573\",\"lineWidth\":2,\"parentID\":15,\"port\":2,\"sid\":[\"\"],\"signalID\":48,\"signalName\":\"Demux11:2\"},\"type\":\"RecordBlkView.Signal\",\"uuid\":\"\"},{\"content\":{\"blockPath\":[],\"channel\":[2],\"dimensions\":[4],\"domain\":\"\",\"lineColor\":\"#ff6929\",\"lineWidth\":2,\"parentID\":17,\"port\":1,\"sid\":[\"\"],\"signalID\":49,\"signalName\":\"Demux10:1\"},\"type\":\"RecordBlkView.Signal\",\"uuid\":\"\"},{\"content\":{\"blockPath\":[],\"channel\":[3],\"dimensions\":[4],\"domain\":\"\",\"lineColor\":\"#b746ff\",\"lineWidth\":2,\"parentID\":17,\"port\":1,\"sid\":[\"\"],\"signalID\":50,\"signalName\":\"Demux10:1\"},\"type\":\"RecordBlkView.Signal\",\"uuid\":\"\"},{\"content\":{\"blockPath\":[],\"channel\":[4],\"dimensions\":[4],\"domain\":\"\",\"lineColor\":\"#64d413\",\"lineWidth\":2,\"parentID\":17,\"port\":1,\"sid\":[\"\"],\"signalID\":51,\"signalName\":\"Demux10:1\"},\"type\":\"RecordBlkView.Signal\",\"uuid\":\"\"},{\"content\":{\"blockPath\":[],\"channel\":[2],\"dimensions\":[4],\"domain\":\"\",\"lineColor\":\"#ff13a6\",\"lineWidth\":2,\"parentID\":19,\"port\":2,\"sid\":[\"\"],\"signalID\":52,\"signalName\":\"Demux10:2\"},\"type\":\"RecordBlkView.Signal\",\"uuid\":\"\"},{\"content\":{\"blockPath\":[],\"channel\":[3],\"dimensions\":[4],\"domain\":\"\",\"lineColor\":\"#fe330a\",\"lineWidth\":2,\"parentID\":19,\"port\":2,\"sid\":[\"\"],\"signalID\":53,\"signalName\":\"Demux10:2\"},\"type\":\"RecordBlkView.Signal\",\"uuid\":\"\"},{\"content\":{\"blockPath\":[],\"channel\":[4],\"dimensions\":[4],\"domain\":\"\",\"lineColor\":\"#22b573\",\"lineWidth\":2,\"parentID\":19,\"port\":2,\"sid\":[\"\"],\"signalID\":54,\"signalName\":\"Demux10:2\"},\"type\":\"RecordBlkView.Signal\",\"uuid\":\"\"},{\"content\":{\"blockPath\":[],\"channel\":[2],\"dimensions\":[4],\"domain\":\"\",\"lineColor\":\"#ff6929\",\"lineWidth\":2,\"parentID\":21,\"port\":1,\"sid\":[\"\"],\"signalID\":55,\"signalName\":\"Demux6:1\"},\"type\":\"RecordBlkView.Signal\",\"uuid\":\"\"},{\"content\":{\"blockPath\":[],\"channel\":[3],\"dimensions\":[4],\"domain\":\"\",\"lineColor\":\"#b746ff\",\"lineWidth\":2,\"parentID\":21,\"port\":1,\"sid\":[\"\"],\"signalID\":56,\"signalName\":\"Demux6:1\"},\"type\":\"RecordBlkView.Signal\",\"uuid\":\"\"},{\"content\":{\"blockPath\":[],\"channel\":[4],\"dimensions\":[4],\"domain\":\"\",\"lineColor\":\"#64d413\",\"lineWidth\":2,\"parentID\":21,\"port\":1,\"sid\":[\"\"],\"signalID\":57,\"signalName\":\"Demux6:1\"},\"type\":\"RecordBlkView.Signal\",\"uuid\":\"\"},{\"content\":{\"blockPath\":[],\"channel\":[2],\"dimensions\":[4],\"domain\":\"\",\"lineColor\":\"#ff13a6\",\"lineWidth\":2,\"parentID\":23,\"port\":2,\"sid\":[\"\"],\"signalID\":58,\"signalName\":\"Demux6:2\"},\"type\":\"RecordBlkView.Signal\",\"uuid\":\"\"},{\"content\":{\"blockPath\":[],\"channel\":[3],\"dimensions\":[4],\"domain\":\"\",\"lineColor\":\"#fe330a\",\"lineWidth\":2,\"parentID\":23,\"port\":2,\"sid\":[\"\"],\"signalID\":59,\"signalName\":\"Demux6:2\"},\"type\":\"RecordBlkView.Signal\",\"uuid\":\"\"},{\"content\":{\"blockPath\":[],\"channel\":[4],\"dimensions\":[4],\"domain\":\"\",\"lineColor\":\"#22b573\",\"lineWidth\":2,\"parentID\":23,\"port\":2,\"sid\":[\"\"],\"signalID\":60,\"signalName\":\"Demux6:2\"},\"type\":\"RecordBlkView.Signal\",\"uuid\":\"\"}]},\"type\":\"RecordBlkView.InputSignals\",\"uuid\":\"\"}],\"packageUris\":[\"http:\\/\\/schema.mathworks.com\\/mf0\\/streamout_blocks\\/R2020a\"],\"version\":\"1.0\"}"  VisualizationBindings="{\"xyplotplugin\":{\"info\":[{\"series\":[{\"bindingParametersList\":[{\"parameter\":\"X-Axis\",\"signalID\":10,\"signalName\":\"Demux8:1(1)\"},{\"parameter\":\"Y-Axis\",\"signalID\":12,\"signalName\":\"Demux8:2(1)\"}],\"seriesID\":0},{\"bindingParametersList\":[{\"parameter\":\"X-Axis\",\"signalID\":37,\"signalName\":\"Demux8:1(2)\"},{\"parameter\":\"Y-Axis\",\"signalID\":40,\"signalName\":\"Demux8:2(2)\"}],\"seriesID\":1},{\"bindingParametersList\":[{\"parameter\":\"X-Axis\",\"signalID\":38,\"signalName\":\"Demux8:1(3)\"},{\"parameter\":\"Y-Axis\",\"signalID\":41,\"signalName\":\"Demux8:2(3)\"}],\"seriesID\":2},{\"bindingParametersList\":[{\"parameter\":\"X-Axis\",\"signalID\":39,\"signalName\":\"Demux8:1(4)\"},{\"parameter\":\"Y-Axis\",\"signalID\":42,\"signalName\":\"Demux8:2(4)\"}],\"seriesID\":3}],\"subplotID\":1}]}}"  CompatibilityTag=XY
  wires:
  Constant6/1 -> State-Space6/1
  Constant7/1 -> State-Space7/1
  Constant8/1 -> State-Space8/1
  Constant9/1 -> State-Space9/1
  State-Space6/1 -> Vector Concatenate/1
  State-Space7/1 -> Vector Concatenate/2
  State-Space8/1 -> Vector Concatenate/3
  State-Space9/1 -> Vector Concatenate/4
  Vector Concatenate/1 -> Demux6/1
  Demux6/1 -> XY Graph7/1
  Demux6/2 -> XY Graph7/2
  Constant12/1 -> State-Space12/1
  Constant10/1 -> State-Space10/1
  Demux7/2 -> XY Graph8/2
  Constant13/1 -> State-Space13/1
  Demux7/1 -> XY Graph8/1
  Constant11/1 -> State-Space11/1
  State-Space12/1 -> Vector Concatenate1/3
  Vector Concatenate1/1 -> Demux7/1
  State-Space13/1 -> Vector Concatenate1/4
  State-Space11/1 -> Vector Concatenate1/2
  State-Space10/1 -> Vector Concatenate1/1
  Constant20/1 -> State-Space20/1
  State-Space19/1 -> Vector Concatenate2/2
  Constant16/1 -> State-Space16/1
  Vector Concatenate2/1 -> Demux8/1
  Constant15/1 -> State-Space15/1
  Demux9/2 -> XY Graph10/2
  State-Space20/1 -> Vector Concatenate2/3
  State-Space16/1 -> Vector Concatenate3/3
  Demux8/1 -> XY Graph9/1
  State-Space17/1 -> Vector Concatenate3/4
  Constant17/1 -> State-Space17/1
  Vector Concatenate3/1 -> Demux9/1
  State-Space18/1 -> Vector Concatenate2/1
  Constant14/1 -> State-Space14/1
  Constant19/1 -> State-Space19/1
  State-Space14/1 -> Vector Concatenate3/1
  Demux9/1 -> XY Graph10/1
  State-Space15/1 -> Vector Concatenate3/2
  Constant18/1 -> State-Space18/1
  Demux8/2 -> XY Graph9/2
  Constant21/1 -> State-Space21/1
  State-Space21/1 -> Vector Concatenate2/4
  Demux11/2 -> XY Graph11/2
  State-Space25/1 -> Vector Concatenate5/4
  Demux10/2 -> XY Graph12/2
  State-Space27/1 -> Vector Concatenate4/2
  State-Space28/1 -> Vector Concatenate4/3
  Constant24/1 -> State-Space24/1
  Vector Concatenate4/1 -> Demux10/1
  Constant29/1 -> State-Space29/1
  Constant28/1 -> State-Space28/1
  Vector Concatenate5/1 -> Demux11/1
  Constant25/1 -> State-Space25/1
  State-Space24/1 -> Vector Concatenate5/3
  Constant23/1 -> State-Space23/1
  Constant22/1 -> State-Space22/1
  Demux10/1 -> XY Graph12/1
  Constant26/1 -> State-Space26/1
  State-Space22/1 -> Vector Concatenate5/1
  State-Space26/1 -> Vector Concatenate4/1
  Constant27/1 -> State-Space27/1
  State-Space29/1 -> Vector Concatenate4/4
  State-Space23/1 -> Vector Concatenate5/2
  Demux11/1 -> XY Graph11/1
